simulink model "untitled1"  (R2025a)
settings: Solver=FixedStepAuto  StartTime=0.0  StopTime=10.0  RelTol=1e-3
settings Model: Creator=nikul  LastModifiedBy=nikul
settings OptimizationCC: DefaultParameterBehavior=Inlined  EnhancedBackFolding=on  PassReuseOutputArgsAs=Individual arguments  ZeroExternalMemoryAtStartup=off  ZeroInternalMemoryAtStartup=off  OptimizeBlockOrder=speed  DifferentSizesBufferReuse=on  OptimizationCustomize=off  EfficientTunableParamExpr=on
settings DebuggingCC: ParameterTunabilityLossMsg=error
settings SFSimCC: MATLABDynamicMemAlloc=off
settings RTWCC: SystemTargetFile=autosar.tlc  GenCodeOnly=on  TemplateMakefile=ert_default_tmf  DataTypeReplacement=CDataTypesFixedWidth  Description=AUTOSAR
settings CodeAppCC: ForceParamTrailComments=on  IgnoreCustomStorageClasses=off  OperatorAnnotations=on  SimulinkDataObjDesc=on  SFDataObjDesc=on  InsertBlockDesc=on
settings STFCustomTargetCC: SystemTargetFile=autosar.tlc  TargetLangStandard=C99 (ISO)  MultiwordLength=256.0  DynamicStringBufferSize=256.0  ParMdlRefBuildCompliant=on  CompOptLevelCompliant=on  IncludeMdlTerminateFcn=off  CombineOutputUpdateFcns=on  SuppressErrorStatus=on  ERTCustomFileBanners=on  SupportNonFinite=off  SupportComplex=off  SupportContinuousTime=off  SupportNonInlinedSFcns=off  RemoveResetFunc=on  MATLABClassNameForMDSCustomization=Simulink.SoftwareTarget.ERTCustomization  AutosarCompliant=on  GRTInterface=off  UseToolchainInfoCompliant=on  LookupTableObjectStructAxisOrder=2,1,3,4,...  LUTObjectStructOrderEvenSpacing=Size,Table,Breakpoints  AutosarCompilerAbstraction=off  AutosarSchemaVersion=R23-11  AutosarMaxShortNameLength=128.0  DisableAUTOSARRoutinesHostLibrary=off  AutosarMatrixIOAsArray=off
settings ERTTargetCC: ExtModeTransport=0.0  ExtModeStaticAlloc=off  ExtModeMexFile=ext_comm  ExtModeIntrfLevel=Level1  ERTCustomFileTemplate=example_file_process.tlc  BooleanTrueId=TRUE  BooleanFalseId=FALSE  TargetLangStandard=C99 (ISO)  ConcurrentExecutionCompliant=off  IncludeMdlTerminateFcn=off  SuppressErrorStatus=on  SupportNonFinite=off  SupportComplex=off  ModelStepFunctionPrototypeControlCompliant=off  CPPClassGenCompliant=off  AutosarCompliant=on  LookupTableObjectStructAxisOrder=2,1,3,4,...  LUTObjectStructOrderEvenSpacing=Size,Table,Breakpoints

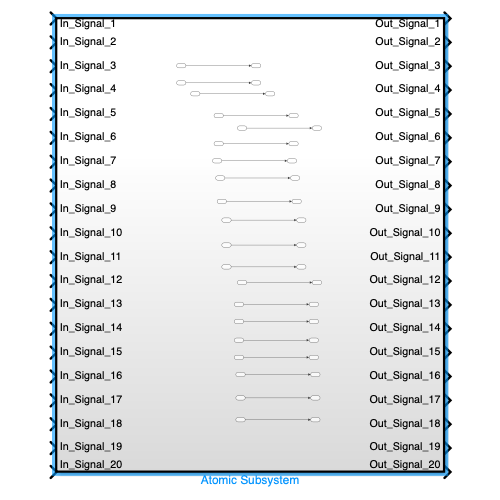
[thumbnail: Simulink's stored preview of the top-level diagram]
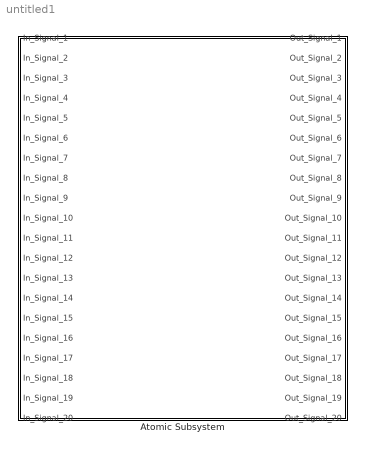
== system untitled1 ==
  Atomic Subsystem : Subsystem  TreatAsAtomicUnit=on

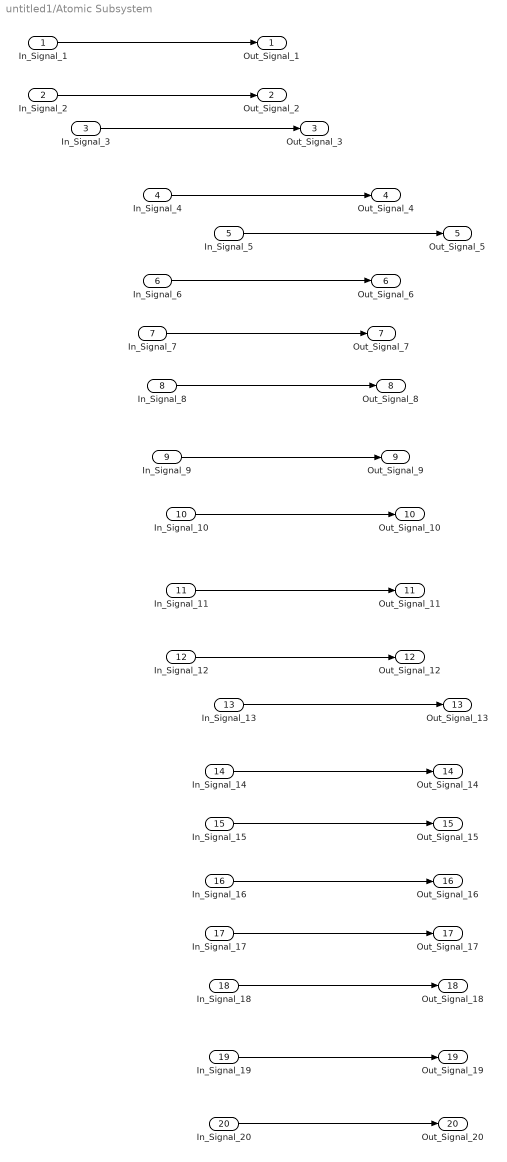
== system untitled1/Atomic Subsystem ==
  In_Signal_1 : Inport
  In_Signal_2 : Inport  Port=2
  In_Signal_3 : Inport  Port=3
  In_Signal_4 : Inport  Port=4
  In_Signal_5 : Inport  Port=5
  In_Signal_6 : Inport  Port=6
  In_Signal_7 : Inport  Port=7
  In_Signal_8 : Inport  Port=8
  In_Signal_9 : Inport  Port=9
  In_Signal_10 : Inport  Port=10
  In_Signal_11 : Inport  Port=11
  In_Signal_12 : Inport  Port=12
  In_Signal_13 : Inport  Port=13
  In_Signal_14 : Inport  Port=14
  In_Signal_15 : Inport  Port=15
  In_Signal_16 : Inport  Port=16
  In_Signal_17 : Inport  Port=17
  In_Signal_18 : Inport  Port=18
  In_Signal_19 : Inport  Port=19
  In_Signal_20 : Inport  Port=20
  Out_Signal_1 : Outport
  Out_Signal_2 : Outport  Port=2
  Out_Signal_3 : Outport  Port=3
  Out_Signal_4 : Outport  Port=4
  Out_Signal_5 : Outport  Port=5
  Out_Signal_6 : Outport  Port=6
  Out_Signal_7 : Outport  Port=7
  Out_Signal_8 : Outport  Port=8
  Out_Signal_9 : Outport  Port=9
  Out_Signal_10 : Outport  Port=10
  Out_Signal_11 : Outport  Port=11
  Out_Signal_12 : Outport  Port=12
  Out_Signal_13 : Outport  Port=13
  Out_Signal_14 : Outport  Port=14
  Out_Signal_15 : Outport  Port=15
  Out_Signal_16 : Outport  Port=16
  Out_Signal_17 : Outport  Port=17
  Out_Signal_18 : Outport  Port=18
  Out_Signal_19 : Outport  Port=19
  Out_Signal_20 : Outport  Port=20
  wires:
  In_Signal_1/1 -> Out_Signal_1/1
  In_Signal_2/1 -> Out_Signal_2/1
  In_Signal_3/1 -> Out_Signal_3/1
  In_Signal_4/1 -> Out_Signal_4/1
  In_Signal_5/1 -> Out_Signal_5/1
  In_Signal_6/1 -> Out_Signal_6/1
  In_Signal_7/1 -> Out_Signal_7/1
  In_Signal_8/1 -> Out_Signal_8/1
  In_Signal_9/1 -> Out_Signal_9/1
  In_Signal_10/1 -> Out_Signal_10/1
  In_Signal_11/1 -> Out_Signal_11/1
  In_Signal_12/1 -> Out_Signal_12/1
  In_Signal_13/1 -> Out_Signal_13/1
  In_Signal_14/1 -> Out_Signal_14/1
  In_Signal_15/1 -> Out_Signal_15/1
  In_Signal_16/1 -> Out_Signal_16/1
  In_Signal_17/1 -> Out_Signal_17/1
  In_Signal_18/1 -> Out_Signal_18/1
  In_Signal_19/1 -> Out_Signal_19/1
  In_Signal_20/1 -> Out_Signal_20/1
